simulink model "sf_sawtooth3"  (R2020a)
settings: Solver=VariableStepAuto  StartTime=0.0  StopTime=10.0  RelTol=1e-3
settings Model: Creator=bzhan  LastModifiedBy=bzhan

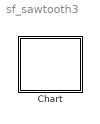
== system sf_sawtooth3 ==
  Chart : Stateflow chart  TreatAsAtomicUnit=on

== stateflow chart sf_sawtooth3/Chart ==
  settings: updateMethod=CONTINUOUS
  state All
    du: x_dot=y;
    state A
      en: y=1;
      du: t_dot=1;
    state B
      en: y=-1;
      du: t_dot=1;
    (default) -> A : {t=1;}
    B -> A : [t>=1]{t=0;}
    A -> B : [t>=1]{t=0;}
  (default) -> All : {x=1;}
  data: y local; t local; x local
  data y settings: updateMethod=SF_CONTINUOUS_TIME_DATA
  data t settings: updateMethod=SF_CONTINUOUS_TIME_DATA
  data x settings: updateMethod=SF_CONTINUOUS_TIME_DATA
